simulink model "uavModel"  (R2017a)
settings: Solver=VariableStepAuto  StartTime=0.0  StopTime=10.0  RelTol=1e-3
settings Model: Creator=tdarrah  LastModifiedBy=tdarrah

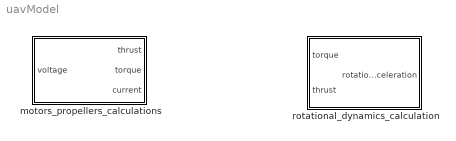
== system uavModel ==
  motors_propellers_calculations : MATLAB Function  TreatAsAtomicUnit=on
  rotational_dynamics_calculation : MATLAB Function  TreatAsAtomicUnit=on

== matlab function uavModel/rotational_dynamics_calculation ==
  data: torque input; rotational_acceleration output; thrust input
function rotational_acceleration = rotational_acceleration_calculation(torque, thrust)
%
% inputs: torque vector
%         thrust vector
%
% output: rotational acceleration (of drone)
%

% moments about each axis (x,y,z) i.e. (pitch, roll, yaw)
moments = [0 0 0];

% rotational acceleration about each axis
rotational_acceleration = [0 0 0];

% moments of inertia empirically derived from sample data
moments_I = [.003, .003, .007];

% pitch
% motor pair A * 1/2 rigid body length - motor pair B * rigid body length
moments(1) = (thrust(3) + thrust(4))*.237/2 - (thrust(1)+thrust(2))*.237/2;
% roll
% motor pair A * 1/2 rigid body length - motor pair B * rigid body length
moments(2) = (thrust(3) + thrust(2))*.237/2 - (thrust(1)+thrust(4))*.237/2;
%yaw
% motor pair A - motor pair B
moments(3) = (torque(4) + torque(2)) - (torque(1)  + torque(3));

for i=1:3
    rotational_acceleration(i) = moments(i) / moments_I(i);
end

== matlab function uavModel/motors_propellers_calculations ==
  data: voltage input; thrust output; torque output; current output
function [thrust, torque, current] = motors_propellers_calculations(voltage)
%
% input: voltage
%
% output: motor torque, 
%         propeller thrust 
%         battery current
%

% rpm constant
KV = 1400;
% per motor
rpm = [0 0 0 0]; 
thrust = [0 0 0 0];
torque = [0 0 0 0];
current = [0 0 0 0];

for i=1:4
    % empirically derived equation given sample data
    rpm(i) = -2.6931*voltage(i)^3 + KV*voltage(i);
    %coefficient of thrust, empirically derived
    coef_t = 2*(10^-15)*rpm(i)^3 - 4*(10^-11)*rpm(i)^2 + 3*(10^-7)*rpm(i) + .1013;
    %thrust = coef_t * density of air * velocity^2 * propeller diameter (m) ^4
    thrust(i) = coef_t*1.225*(rpm(i)/60)^2*.2^4;
    % empirically derived
    torque(i) = 4*(10^-14)*rpm(i)^3 +  8*(10^-12)*rpm(i)^2 + 3*(10^-6)*rpm(i);
    % current = rpm constant * torque
    current(i) = KV*torque(i);
end
